simulink model "DAB_Converter_D2"  (R2024a)
settings: Solver=VariableStepAuto  StartTime=0.0  StopTime=0.1  RelTol=1e-3
libraries: spsMosfetLib x8, spsCurrentMeasurementLib x3, spsVoltageMeasurementLib x3, spsDCVoltageSourceLib x2, spsMeanLib x2, spsLinearTransformerLib x1, spsRMSLib x1, spsSeriesRLCBranchLib x1, sps_lib x1
settings Model: Creator=abhik  LastModifiedBy=abhik

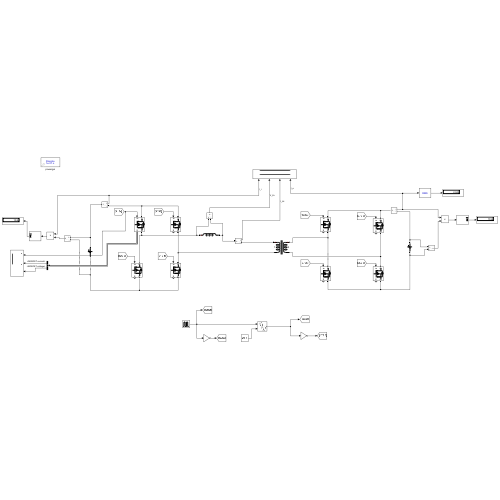
[thumbnail: Simulink's stored preview of the top-level diagram]
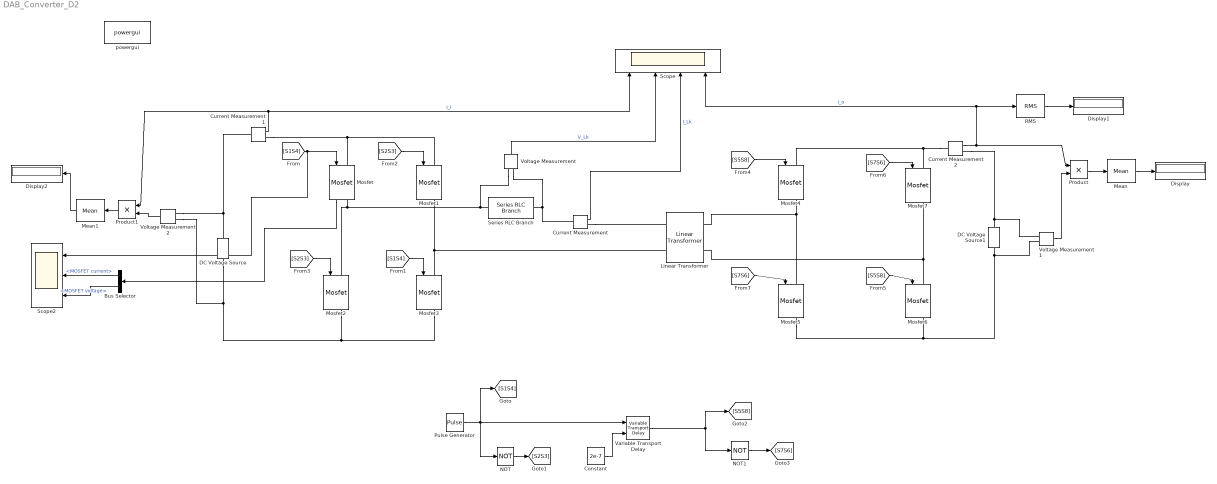
== system DAB_Converter_D2 ==
  Bus Selector : BusSelector  OutputSignals=MOSFET current,MOSFET voltage
  Constant : Constant  Value=2e-7
  Current Measurement : spsCurrentMeasurementLib/Current Measurement  PhasorSimulation=off  OutputType=Complex  PSBequivalent=0
  Current Measurement1 : spsCurrentMeasurementLib/Current Measurement  PhasorSimulation=off  OutputType=Complex  PSBequivalent=0
  Current Measurement2 : spsCurrentMeasurementLib/Current Measurement  PhasorSimulation=off  OutputType=Complex  PSBequivalent=0
  DC Voltage Source : spsDCVoltageSourceLib/DC Voltage Source  Amplitude=48  Measurements=None
  DC Voltage Source1 : spsDCVoltageSourceLib/DC Voltage Source  Amplitude=400  Measurements=None
  Display : Display
  Display1 : Display
  Display2 : Display
  Linear Transformer : spsLinearTransformerLib/Linear Transformer  UNITS=SI  NominalPower=[ 1000 100e3]  winding1=[48 0 0]  winding2=[384 0 0]  ThreeWindings=off  winding3=[3.15e+05 0.7938 0.084225]  RmLm=[1.0804e+06 2866]  Measurements=None  DataType=on
  Mean : spsMeanLib/Mean  Freq=60  Vinit=0  Ts=0
  Mean1 : spsMeanLib/Mean  Freq=60  Vinit=0  Ts=0
  Mosfet : spsMosfetLib/Mosfet  Ron=0.0001  Lon=0  Rd=1e-4  Vfd=0  IC=0  Rs=1e6  Cs=1000e-12  Measurements=on
  Mosfet1 : spsMosfetLib/Mosfet  Ron=0.0001  Lon=0  Rd=1e-4  Vfd=0  IC=0  Rs=1e6  Cs=1000e-12  Measurements=on
  Mosfet2 : spsMosfetLib/Mosfet  Ron=0.001  Lon=0  Rd=1e-4  Vfd=0  IC=0  Rs=1e6  Cs=1000e-12  Measurements=on
  Mosfet3 : spsMosfetLib/Mosfet  Ron=0.001  Lon=0  Rd=1e-4  Vfd=0  IC=0  Rs=1e6  Cs=1000e-12  Measurements=on
  Mosfet{4..7} (4 alike) : spsMosfetLib/Mosfet  Ron=0.0001  Lon=0  Rd=1e-4  Vfd=0  IC=0  Rs=1e6  Cs=100e-12  Measurements=on
  NOT : Logic  Operator=NOT  IconShape=distinctive  AllPortsSameDT=off  OutDataTypeStr=boolean
  NOT1 : Logic  Operator=NOT  IconShape=distinctive  AllPortsSameDT=off  OutDataTypeStr=boolean
  Product : Product
  Product1 : Product
  Pulse Generator : DiscretePulseGenerator  PulseType=Time based  Period=1e-5  PulseWidth=50
  RMS : spsRMSLib/RMS  TrueRMS=on  Freq=60  RMSInit=120  Ts=0
  Scope : Scope  NumInputPorts=4
  Scope2 : Scope  NumInputPorts=3
  Series RLC Branch : spsSeriesRLCBranchLib/Series RLC Branch  LConnTagsString=__new0  RConnTagsString=__new0  BranchType=L  Resistance=1  Inductance=0.44e-6  SetiL0=off  InitialCurrent=0  Capacitance=1e-6  Setx0=off  InitialVoltage=0  Measurements=None
  Variable Transport Delay : VariableTransportDelay  MaximumDelay=10
  Voltage Measurement : spsVoltageMeasurementLib/Voltage Measurement  PhasorSimulation=off  OutputType=Complex  PSBequivalent=0
  Voltage Measurement1 : spsVoltageMeasurementLib/Voltage Measurement  PhasorSimulation=off  OutputType=Complex  PSBequivalent=0
  Voltage Measurement2 : spsVoltageMeasurementLib/Voltage Measurement  PhasorSimulation=off  OutputType=Complex  PSBequivalent=0
  powergui : sps_lib/powergui  Priority=1  SimulationMode=Discrete  SampleTime=1e-7  frequency=60  Iterations=50  frequencyindice=0  Pbase=100e6  ErrMax=1e-4  UnitsV=kV  UnitsW=MW  buscounter=0  FunctionMessages=off  echomessages=off  EnableUseOfTLC=off  CurrentSourceSwitches=off  DisableSnubberDevices=off  DisableRonSwitches=off  DisableVfSwitches=off  DisplayEquations=off  AutomaticDiscreteSolvers=off  SolverType=Tustin/Backward Euler (TBE)  Interpol=off  ExternalGateDelay=off  methode=off  Ts=100  x0status=blocks  SPID=on  SwTol=0  HookPort=off  NonlinearTolerance=1e-4  nMaxIteration=100  ContinueOnMaxIteration=off  RestoreLinks=warning  ResistiveCurrentMeasurement=off  Frange=[0:2:500]  Ylog=off  Xlog=on  ShowGrid=off  save=off  variable=ZData  structure=0  ZoomFFT=off  StartTime=0.0  cycles=1  DisplayStyle=1  fundamental=60  FreqAxis=off  MaxFrequency=1000  frequencyindicesteady=1  RmsSteady=1  display=off
  wires:
  Current Measurement2/1 -> Product/1, RMS/1, Scope/4  "I_o"
  [S2S3] -> Mosfet2/1
  [S7S6] -> Mosfet5/1
  Current Measurement1/1 -> Scope/1, Product1/1  "I_i"
  [S5S8] -> Mosfet6/1
  [S7S6] -> Mosfet7/1
  [S5S8] -> Mosfet4/1
  NOT1/1 -> [S7S6]
  [S1S4] -> Mosfet3/1
  Voltage Measurement/1 -> Scope/2  "V_Lk"
  [S2S3] -> Mosfet1/1
  Pulse Generator/1 -> [S1S4], Variable Transport Delay/1, NOT/1
  Current Measurement/1 -> Scope/3  "I_Lk"
  [S1S4] -> Mosfet/1, Scope2/1
  NOT/1 -> [S2S3]
  Voltage Measurement1/1 -> Product/2
  Product/1 -> Mean/1
  Mean/1 -> Display/1
  RMS/1 -> Display1/1
  Constant/1 -> Variable Transport Delay/2
  Variable Transport Delay/1 -> [S5S8], NOT1/1
  Voltage Measurement2/1 -> Product1/2
  Product1/1 -> Mean1/1
  Mean1/1 -> Display2/1
  Mosfet/1 -> Bus Selector/1
  Bus Selector/1 -> Scope2/2  "<MOSFET current>"
  Bus Selector/2 -> Scope2/3  "<MOSFET voltage>"
  connections:
  Current Measurement2/LConn1 -- Mosfet4/LConn1 -- Mosfet7/LConn1
  Mosfet1/RConn1 -- Linear Transformer/LConn2 -- Mosfet3/LConn1
  Mosfet/LConn1 -- Mosfet1/LConn1 -- Current Measurement1/RConn1
  Linear Transformer/RConn2 -- Mosfet7/RConn1 -- Mosfet6/LConn1
  Mosfet6/RConn1 -- Voltage Measurement1/LConn2 -- DC Voltage Source1/LConn1 -- Mosfet5/RConn1
  Series RLC Branch/RConn1 -- Current Measurement/LConn1 -- Voltage Measurement/LConn2
  Mosfet4/RConn1 -- Mosfet5/LConn1 -- Linear Transformer/RConn1
  Mosfet/RConn1 -- Mosfet2/LConn1 -- Series RLC Branch/LConn1 -- Voltage Measurement/LConn1
  Mosfet2/RConn1 -- Voltage Measurement2/LConn2 -- DC Voltage Source/LConn1 -- Mosfet3/RConn1
  Current Measurement/RConn1 -- Linear Transformer/LConn1
  Current Measurement2/RConn1 -- Voltage Measurement1/LConn1 -- DC Voltage Source1/RConn1
  DC Voltage Source/RConn1 -- Current Measurement1/LConn1 -- Voltage Measurement2/LConn1
